simulink model "Engine"  (R2019a)
settings: Solver=VariableStepAuto  StartTime=0.0  StopTime=10.0  RelTol=1e-3
values from neighbouring files (symbols this model uses):
  D = P2B*(CG-RP)    [getAeroCoeff.m]
  Par = Init_Propulsion    [getEngData.m]
libraries: sharedutil x1
settings Model: Creator=haberdav  LastModifiedBy=haberdav
settings DataIOCC: SaveFormat=Array

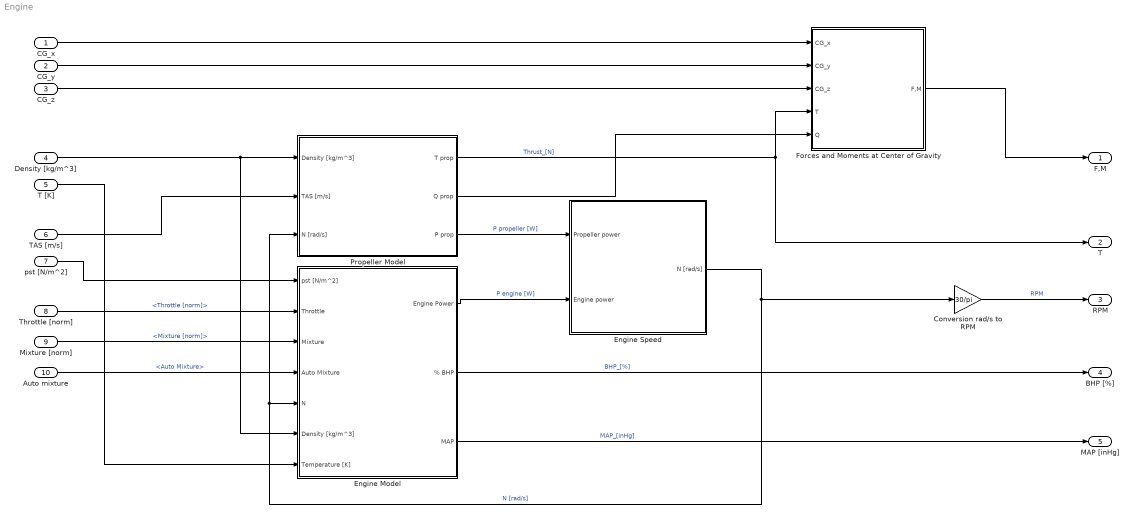
== system Engine ==
  CG_x : Inport
  CG_y : Inport  Port=2
  CG_z : Inport  Port=3
  Density [kg/m^3] : Inport  Port=4
  "T [K] " : Inport  Port=5
  TAS [m/s] : Inport  Port=6
  pst [N/m^2] : Inport  Port=7
  Throttle [norm] : Inport  Port=8
  Mixture [norm] : Inport  Port=9
  Auto mixture : Inport  Port=10
  Conversion rad/s to RPM : Gain  Gain=30/pi
  Engine Model : Subsystem
  Engine Speed : Subsystem
  Forces and Moments at Center of Gravity : Subsystem
  Propeller Model : Subsystem
  F,M : Outport
  T : Outport  Port=2
  RPM : Outport  Port=3
  BHP [%] : Outport  Port=4
  MAP [inHg] : Outport  Port=5
  wires:
  CG_x/1 -> Forces and Moments at Center of Gravity/1(CG_x)
  pst [N/m^2]/1 -> Engine Model/1(pst [N/m^2])
  CG_z/1 -> Forces and Moments at Center of Gravity/3(CG_z)
  "T [K] "/1 -> Engine Model/7(Temperature [K])
  CG_y/1 -> Forces and Moments at Center of Gravity/2(CG_y)
  Mixture [norm]/1 -> Engine Model/3(Mixture)  "<Mixture [norm]>"
  Density [kg/m^3]/1 -> Engine Model/6(Density [kg/m^3]), Propeller Model/1(Density [kg/m^3])
  Auto mixture/1 -> Engine Model/4(Auto Mixture)  "<Auto Mixture>"
  Engine Model/1(Engine Power) -> Engine Speed/2(Engine power)  "P engine [W]"
  Engine Speed/1(N [rad/s]) -> Propeller Model/3(N [rad/s]), Engine Model/5(N), Conversion rad/s to RPM/1  "N [rad/s]"
  Propeller Model/2(Q prop) -> Forces and Moments at Center of Gravity/5(Q)
  TAS [m/s]/1 -> Propeller Model/2(TAS [m/s])
  Throttle [norm]/1 -> Engine Model/2(Throttle)  "<Throttle [norm]>"
  Propeller Model/3(P prop) -> Engine Speed/1(Propeller power)  "P propeller [W]"
  Propeller Model/1(T prop) -> T/1, Forces and Moments at Center of Gravity/4(T)  "Thrust_[N]"
  Engine Model/3(MAP) -> MAP [inHg]/1  "MAP_[inHg]"
  Conversion rad/s to RPM/1 -> RPM/1  "RPM"
  Engine Model/2(% BHP) -> BHP [%]/1  "BHP_[%]"
  Forces and Moments at Center of Gravity/1(F,M) -> F,M/1

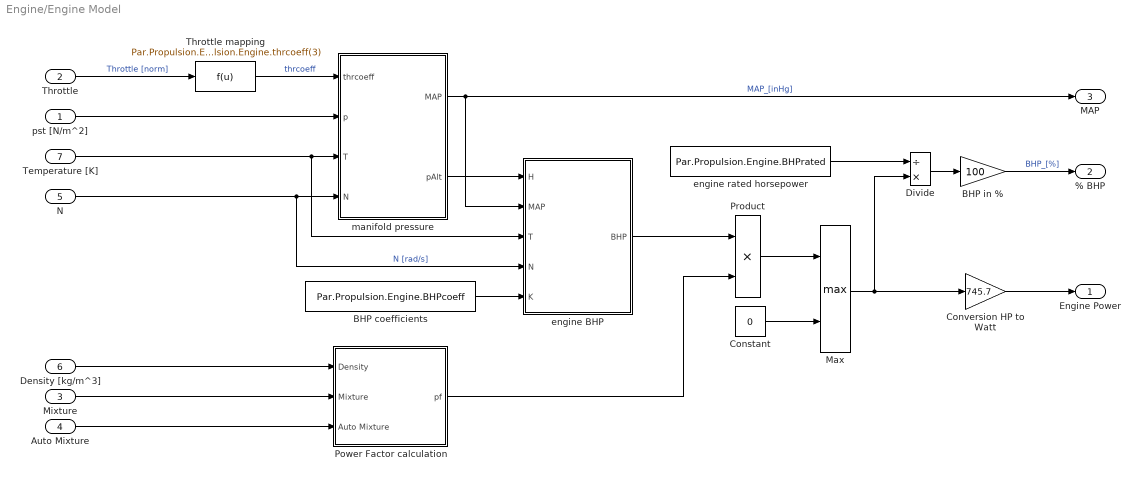
== system Engine/Engine Model ==
  pst [N/m^2] : Inport
  Throttle : Inport  Port=2
  Mixture : Inport  Port=3
  Auto Mixture : Inport  Port=4
  N : Inport  Port=5
  Density [kg/m^3] : Inport  Port=6
  Temperature [K] : Inport  Port=7
  BHP coefficients : Constant  Value=Par.Propulsion.Engine.BHPcoeff
  BHP in % : Gain  Gain=100
  Constant : Constant  Value=0
  Conversion HP to Watt : Gain  Gain=745.7
  Divide : Product  Inputs=/*
  Max : MinMax  Function=max  Inputs=2
  Power Factor calculation : Subsystem
  Product : Product
  Throttle mapping : Fcn  Expr=Par.Propulsion.Engine.thrcoeff(1)*u^2 + Par.Propulsion.Engine.thrcoeff(2)*u + Par.Propulsion.Engine.thrcoeff(3)
  engine BHP : MATLAB Function  TreatAsAtomicUnit=on
  engine rated horsepower : Constant  Value=Par.Propulsion.Engine.BHPrated
  manifold pressure : MATLAB Function  TreatAsAtomicUnit=on  mask{R=Par.Environment.Atmosphere.R, Vd=Par.Propulsion.Engine.Vd, etaV=Par.Propulsion.Engine.etaV, k=Par.Propulsion.Engine.mthcoeff, g=Par.Environment.Atmosphere.g_n, ga0=Par.Environment.Atmosphere.ga_0}
      mask prompts: R "Gas constant for air [J/kg/K]"; Vd "Engine displaced volume [m^3]"; etaV "Engine volumetric efficiency [-]"; k "Full throttle air mass flow coefficients"; g "Gravity acceleration [m/s^2]"; ga0 "Temperature gradient for troposphere [K/m]"
  Engine Power : Outport
  % BHP : Outport  Port=2
  MAP : Outport  Port=3
  wires:
  manifold pressure/2(pAlt) -> engine BHP/1(H)
  Constant/1 -> Max/2
  Product/1 -> Max/1
  Throttle mapping/1 -> manifold pressure/1(thrcoeff)  "thrcoeff"
  Density [kg/m^3]/1 -> Power Factor calculation/1(Density)
  Conversion HP to Watt/1 -> Engine Power/1
  Max/1 -> Conversion HP to Watt/1, Divide/2
  BHP in %/1 -> % BHP/1  "BHP_[%]"
  manifold pressure/1(MAP) -> MAP/1, engine BHP/2(MAP)  "MAP_[inHg]"
  Temperature [K]/1 -> manifold pressure/3(T), engine BHP/3(T)
  Throttle/1 -> Throttle mapping/1  "Throttle [norm]"
  N/1 -> manifold pressure/4(N), engine BHP/4(N)  "N [rad/s]"
  engine rated horsepower/1 -> Divide/1
  Divide/1 -> BHP in %/1
  BHP coefficients/1 -> engine BHP/5(K)
  engine BHP/1(BHP) -> Product/1
  Mixture/1 -> Power Factor calculation/2(Mixture)
  Power Factor calculation/1(pf) -> Product/2
  Auto Mixture/1 -> Power Factor calculation/3(Auto Mixture)
  pst [N/m^2]/1 -> manifold pressure/2(p)

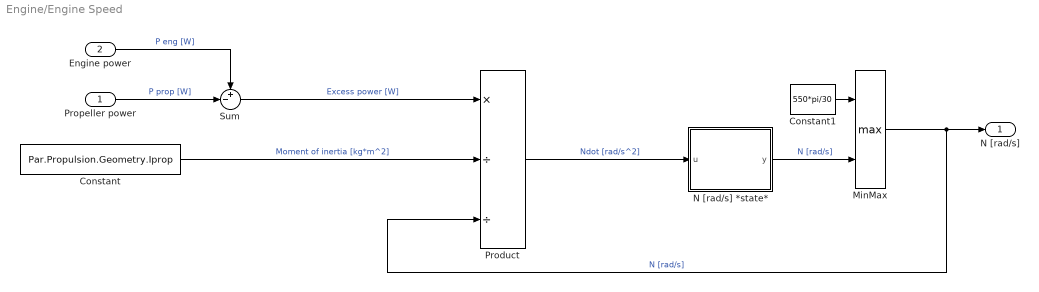
== system Engine/Engine Speed ==
  Propeller power : Inport
  Engine power : Inport  Port=2
  Constant : Constant  Value=Par.Propulsion.Geometry.Iprop
  Constant1 : Constant  Value=550*pi/30
  MinMax : MinMax  Function=max  Inputs=2
  N [rad/s] *state* : Subsystem  mask(Generic Integrator for Aircraft States){T=Par.Sim.Ts.EOM, IC=Par.IC.N0}
      mask prompts: T "Sample Time"; IC "Initial Condition"
      mask Display:
      | patch([.2,.8,.8,.2,.2],[.2,.2,.8,.8,.2],[.75,.75,.75])
      | fprintf('1\ns')
      | plot([.45,.55],[.5,.5])
      | text(.55,.1,sprintf('T=%0.3g',T))
  Product : Product  Inputs=*//
  Sum : Sum  Inputs=+-|
  N [rad/s] : Outport
  wires:
  Constant1/1 -> MinMax/1
  MinMax/1 -> N [rad/s]/1, Product/3  "N [rad/s]"
  N [rad/s] *state*/1(y) -> MinMax/2  "N [rad/s]"
  Engine power/1 -> Sum/1  "P eng [W]"
  Propeller power/1 -> Sum/2  "P prop [W]"
  Sum/1 -> Product/1  "Excess power [W]"
  Constant/1 -> Product/2  "Moment of inertia [kg*m^2]"
  Product/1 -> N [rad/s] *state*/1(u)  "Ndot [rad/s^2]"

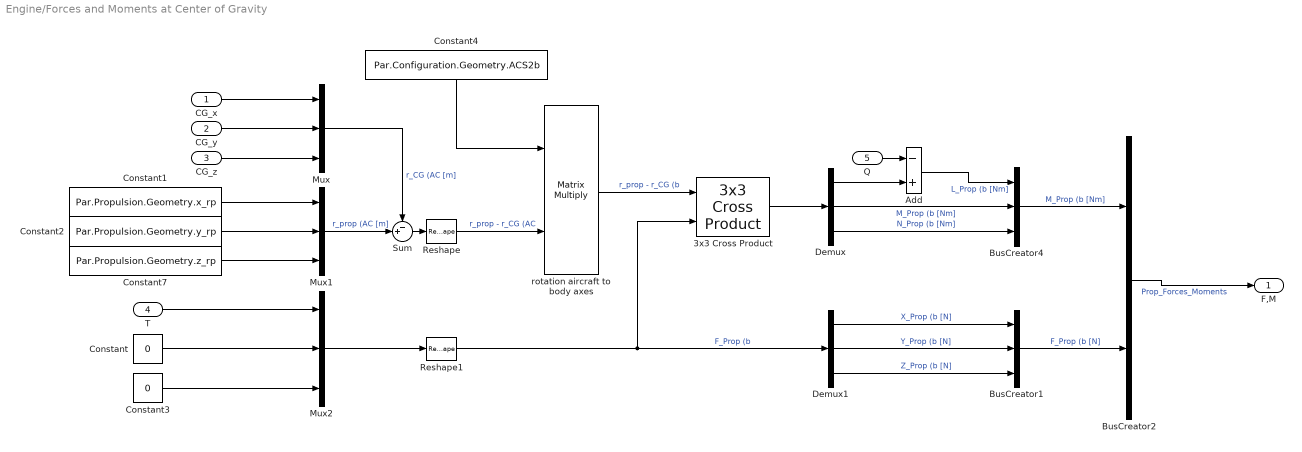
== system Engine/Forces and Moments at Center of Gravity ==
  CG_x : Inport
  CG_y : Inport  Port=2
  CG_z : Inport  Port=3
  T : Inport  Port=4
  Q : Inport  Port=5
  3x3 Cross Product : sharedutil/3x3 Cross Product  aMode=aMode
      settings: SourceProductBaseCode=AE
  Add : Sum  Inputs=-+
  BusCreator1 : BusCreator  Inputs=3
  BusCreator2 : BusCreator  Inputs=2
  BusCreator4 : BusCreator  Inputs=3
  Constant : Constant  Value=0
  Constant1 : Constant  Value=Par.Propulsion.Geometry.x_rp  VectorParams1D=off
  Constant2 : Constant  Value=Par.Propulsion.Geometry.y_rp  VectorParams1D=off
  Constant3 : Constant  Value=0
  Constant4 : Constant  Value=Par.Configuration.Geometry.ACS2b  VectorParams1D=off
  Constant7 : Constant  Value=Par.Propulsion.Geometry.z_rp  VectorParams1D=off
  Demux : Demux  Outputs=3
  Demux1 : Demux  Outputs=3
  Mux : Mux  Inputs=3
  Mux1 : Mux  Inputs=3
  Mux2 : Mux  Inputs=3
  Reshape : Reshape  OutputDimensionality=Column vector (2-D)
  Reshape1 : Reshape  OutputDimensionality=Column vector (2-D)
  Sum : Sum  Inputs=-+|
  rotation aircraft to body axes : Product  Multiplication=Matrix(*)
  F,M : Outport
  wires:
  Reshape1/1 -> 3x3 Cross Product/2, Demux1/1  "F_Prop (b"
  Reshape/1 -> rotation aircraft to body axes/2  "r_prop - r_CG (AC"
  rotation aircraft to body axes/1 -> 3x3 Cross Product/1  "r_prop - r_CG (b"
  Constant4/1 -> rotation aircraft to body axes/1
  Sum/1 -> Reshape/1
  Constant3/1 -> Mux2/3
  Constant/1 -> Mux2/2
  T/1 -> Mux2/1
  Demux/1 -> Add/2
  Add/1 -> BusCreator4/1  "L_Prop (b [Nm]"
  Demux1/1 -> BusCreator1/1  "X_Prop (b [N]"
  Demux1/3 -> BusCreator1/3  "Z_Prop (b [N]"
  Demux/3 -> BusCreator4/3  "N_Prop (b [Nm]"
  Demux/2 -> BusCreator4/2  "M_Prop (b [Nm]"
  Mux2/1 -> Reshape1/1
  Mux1/1 -> Sum/2  "r_prop (AC [m]"
  Mux/1 -> Sum/1  "r_CG (AC [m]"
  CG_z/1 -> Mux/3
  CG_y/1 -> Mux/2
  CG_x/1 -> Mux/1
  Constant7/1 -> Mux1/3
  Constant2/1 -> Mux1/2
  Constant1/1 -> Mux1/1
  Demux1/2 -> BusCreator1/2  "Y_Prop (b [N]"
  Q/1 -> Add/1
  3x3 Cross Product/1 -> Demux/1
  BusCreator1/1 -> BusCreator2/2  "F_Prop (b [N]"
  BusCreator4/1 -> BusCreator2/1  "M_Prop (b [Nm]"
  BusCreator2/1 -> F,M/1  "Prop_Forces_Moments"

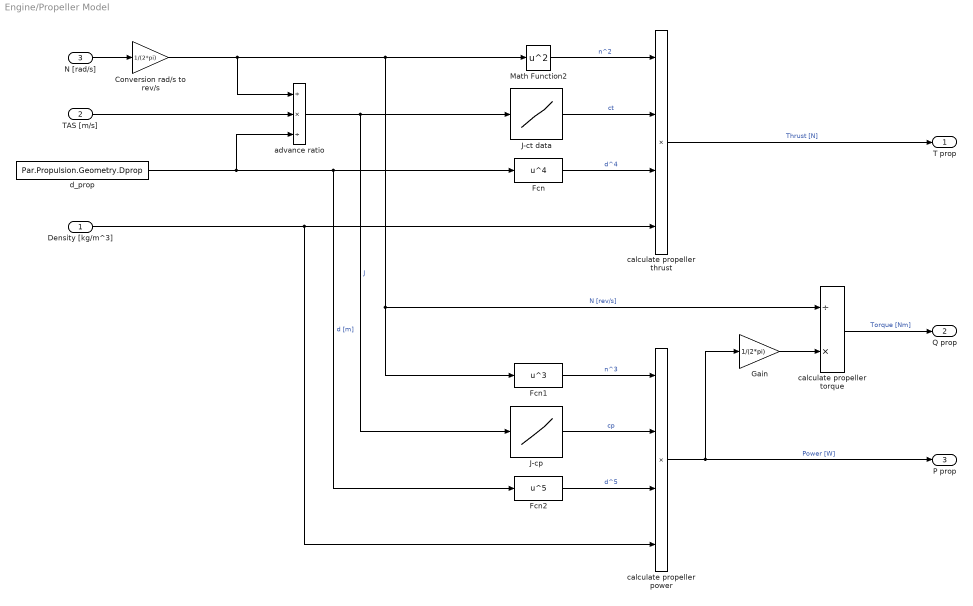
== system Engine/Propeller Model ==
  Density [kg/m^3] : Inport
  TAS [m/s] : Inport  Port=2
  N [rad/s] : Inport  Port=3
  Conversion rad/s to rev/s : Gain  Gain=1/(2*pi)
  Fcn : Fcn  Expr=u^4
  Fcn1 : Fcn  Expr=u^3
  Fcn2 : Fcn  Expr=u^5
  Gain : Gain  Gain=1/(2*pi)
  J-cp : Lookup_n-D  NumberOfTableDimensions=1  BreakpointsForDimension1=Par.Propulsion.Prop.J  Table=Par.Propulsion.Prop.c_p  InternalRulePriority=Speed  RndMeth=Simplest  InputSameDT=on
  J-ct data : Lookup_n-D  NumberOfTableDimensions=1  BreakpointsForDimension1=Par.Propulsion.Prop.J  Table=Par.Propulsion.Prop.c_t  InternalRulePriority=Speed  RndMeth=Simplest  InputSameDT=on
  Math Function2 : Math  Operator=square  SaturateOnIntegerOverflow=on
  advance ratio : Product  Inputs=/*/
  calculate propeller power : Product  Inputs=4  OutMin=0
  calculate propeller thrust : Product  Inputs=4  OutMin=0
  calculate propeller torque : Product  Inputs=/*
  d_prop : Constant  Value=Par.Propulsion.Geometry.Dprop
  T prop : Outport
  Q prop : Outport  Port=2
  P prop : Outport  Port=3
  wires:
  calculate propeller thrust/1 -> T prop/1  "Thrust [N]"
  Conversion rad/s to rev/s/1 -> advance ratio/1, Fcn1/1, calculate propeller torque/1, Math Function2/1  "N [rev/s]"
  J-ct data/1 -> calculate propeller thrust/2  "ct"
  Math Function2/1 -> calculate propeller thrust/1  "n^2"
  advance ratio/1 -> J-ct data/1, J-cp/1  "J"
  d_prop/1 -> Fcn2/1, Fcn/1, advance ratio/3  "d [m]"
  Fcn/1 -> calculate propeller thrust/3  "d^4"
  TAS [m/s]/1 -> advance ratio/2
  Density [kg/m^3]/1 -> calculate propeller power/4, calculate propeller thrust/4
  Fcn1/1 -> calculate propeller power/1  "n^3"
  J-cp/1 -> calculate propeller power/2  "cp"
  Fcn2/1 -> calculate propeller power/3  "d^5"
  calculate propeller power/1 -> Gain/1, P prop/1  "Power [W]"
  Gain/1 -> calculate propeller torque/2
  calculate propeller torque/1 -> Q prop/1  "Torque [Nm]"
  N [rad/s]/1 -> Conversion rad/s to rev/s/1

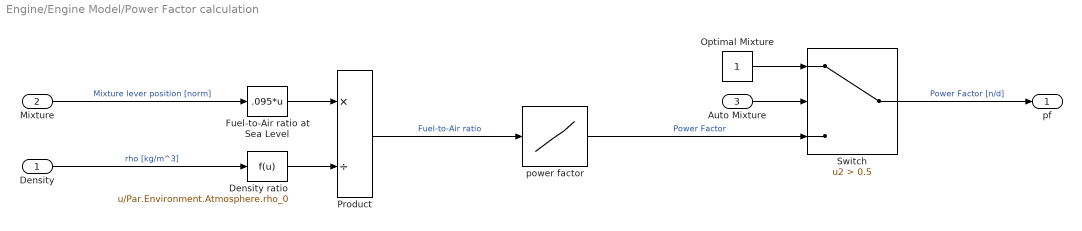
== system Engine/Engine Model/Power Factor calculation ==
  Density : Inport
  Mixture : Inport  Port=2
  Auto Mixture : Inport  Port=3
  Density ratio : Fcn  Expr=u/Par.Environment.Atmosphere.rho_0
  Fuel-to-Air ratio at Sea Level : Fcn  Expr=.095*u
  Optimal Mixture : Constant
  Product : Product  Inputs=*/
  Switch : Switch  Criteria=u2 > Threshold  Threshold=0.5
  power factor : Lookup_n-D  NumberOfTableDimensions=1  BreakpointsForDimension1=Par.Propulsion.Engine.FAratio  Table=Par.Propulsion.Engine.pf  InternalRulePriority=Speed  RndMeth=Simplest  InputSameDT=on
  pf : Outport
  wires:
  Product/1 -> power factor/1  "Fuel-to-Air ratio"
  Density/1 -> Density ratio/1  "rho [kg/m^3]"
  Density ratio/1 -> Product/2
  Mixture/1 -> Fuel-to-Air ratio at Sea Level/1  "Mixture lever position [norm]"
  Fuel-to-Air ratio at Sea Level/1 -> Product/1
  power factor/1 -> Switch/3  "Power Factor"
  Switch/1 -> pf/1  "Power Factor [n/d]"
  Auto Mixture/1 -> Switch/2
  Optimal Mixture/1 -> Switch/1

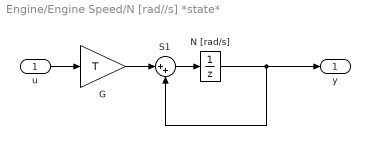
== system Engine/Engine Speed/N [rad//s] *state* ==
  u : Inport
  G : Gain  Gain=T  SaturateOnIntegerOverflow=on  OutDataTypeStr=Inherit: Same as input  ParamDataTypeStr=Inherit: Same as input
  N [rad/s] : UnitDelay  InitialCondition=IC  SampleTime=T  HasFrameUpgradeWarning=on
  S1 : Sum  Inputs=|++  SaturateOnIntegerOverflow=on
  y : Outport
  wires:
  S1/1 -> N [rad/s]/1
  u/1 -> G/1
  N [rad/s]/1 -> S1/2, y/1
  G/1 -> S1/1

== matlab function Engine/Engine Model/engine BHP ==
  data: H input; MAP input; T input; N input; BHP output; K input
function BHP = engBHPcalc(H,MAP,T,N,K)

% Units conversion
H = H/0.3048; % pressure altitude: m to ft
T = (T - 273.15)*9/5 + 32; % temperature: K to °F
RPM = N*30/pi; % engine speed: rad/s to RPM

% linearly extrapolate engine BHP if RPM is outside the range considered in
% engine performance charts
if RPM < 2000
        BHP = SmithDreier(MAP,H,T,2000,K)*RPM/2000; 
    else
        BHP = SmithDreier(MAP,H,T,RPM,K);
end
    
return

%% Engine brake horsepower calculation
function BHPE = SmithDreier(MAP,H,T,RPM,K)
% Temperature ratio
theta = (460 + T)/519;

% Pressure ratio
delta = (1 - 0.689e-5*H).^5.256;

% Equation (1)
BHPA = K(1) + K(2)*RPM + K(3)*MAP + K(4)*RPM.*MAP + K(5)*MAP.^2 + K(6)*RPM.*MAP.^2;

% Equation (2)
BHPB = K(7) + K(8)*RPM + K(9)*MAP + K(10)*MAP.*RPM;

% Equation (3)
BHPSL = K(11) + K(12)*RPM + K(13)*RPM.^2;

% Equation (4)
sigmaA = 0.117 + 0.883*BHPA./BHPSL;

% Equation (5)
sigmaD = delta./theta;

% Equation (6)
BHPD = BHPB + (BHPA - BHPB).*(1 - sigmaD)./(1 - sigmaA);

% Equation (7)
BHPE = BHPD.*sqrt((1 - 0.689e-5*H)./theta);

return

== matlab function Engine/Engine Model/manifold pressure ==
  data: thrcoeff input; p input; T input; N input; MAP output; k parameter; R parameter; Vd parameter; etaV parameter; pAlt output; g parameter; ga0 parameter
function [MAP,pAlt] = engMAPcalc(thrcoeff,p,T,N,k,R,Vd,etaV,g, ga0)

% Calculate pressure altitude
p0 = 101325; % Standard pressure at Sea Level [Pa]
T0 = 288.15; % Standard temperature at Sea Level [Pa]
pAlt = -(1 - (p/p0)^(-ga0*R/g))*T0/ga0; % Pressure altitude [m]

% Unit conversion: rad/s to rev/s
N = N/(2*pi);

% Air mass flow at full throttle
mthft = N*(k(1) + k(2)*N + k(3)*pAlt + k(4)*N*pAlt + k(5)*pAlt^2 + k(6)*N*pAlt^2);

% Air mass flow at part throttle
mthpt = mthft*thrcoeff;

% manifold pressure [Pa]
MAP = 2*T*R*mthpt/(N*Vd*etaV);

% unit conversion: Pa to inHg
MAP = MAP/3386.39;
